simulink model "TestAllDynamicModelsRealForce"  (R2022b)
settings: Solver=FixedStepAuto  StartTime=0.0  StopTime=137  FixedStep=simulator.TimeStep  RelTol=1e-3
undefined symbols (not defined in the file): simulator
settings Model: Creator=At  LastModifiedBy=ateay
settings SolverCC: ConcurrentTasks=on  AlgebraicLoopSolver=TrustRegion  InsertRTBMode=Never (minimum delay)
settings DataIOCC: ReturnWorkspaceOutputs=off
settings DebuggingCC: UnconnectedInputMsg=warning  UnconnectedOutputMsg=warning  UnconnectedLineMsg=warning  SFMachineParentedDataDiag=warning  ArithmeticOperatorsInVariantConditions=warning
settings ModelReferenceCC: EnableRefExpFcnMdlSchedulingChecks=on
settings SFSimCC: SimUseLocalCustomCode=off  CustomCodeUndefinedFunction=UseInterfaceOnly
settings RTWCC: RTWUseLocalCustomCode=off
settings CodeAppCC: StateflowObjectComments=on

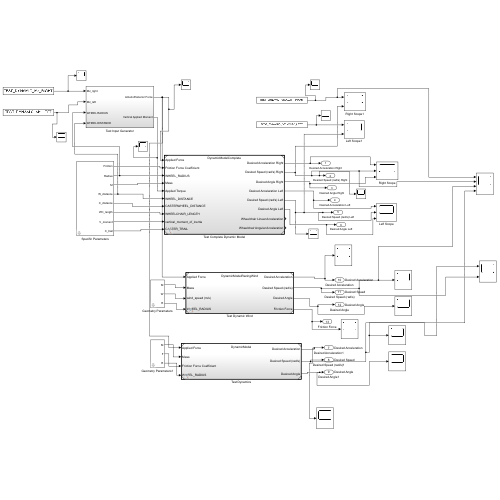
[thumbnail: Simulink's stored preview of the top-level diagram]
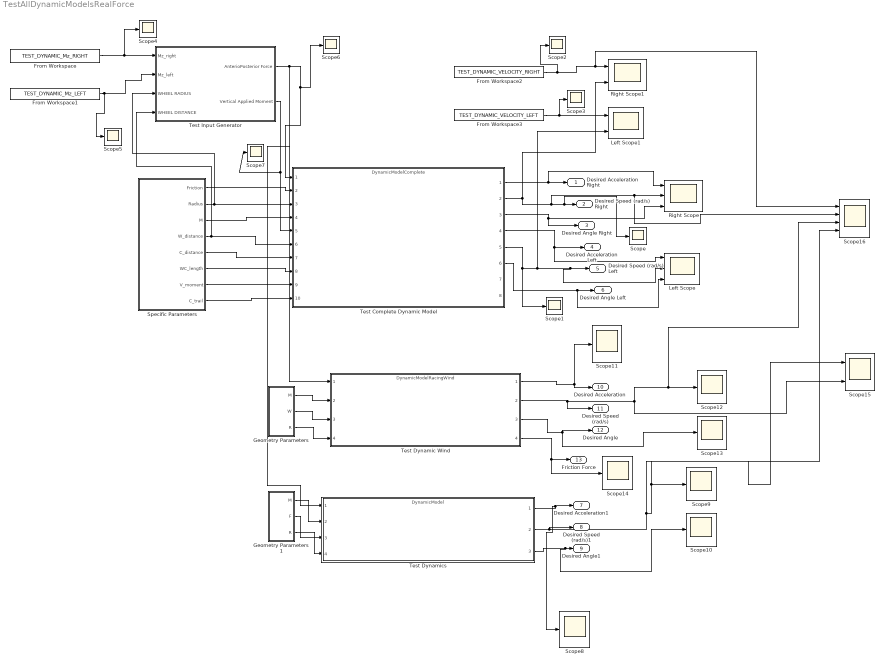
== system TestAllDynamicModelsRealForce ==
  From Workspace : FromWorkspace  VariableName=TEST_DYNAMIC_Mz_RIGHT
  From Workspace1 : FromWorkspace  VariableName=TEST_DYNAMIC_Mz_LEFT
  From Workspace2 : FromWorkspace  VariableName=TEST_DYNAMIC_VELOCITY_RIGHT
  From Workspace3 : FromWorkspace  VariableName=TEST_DYNAMIC_VELOCITY_LEFT
  Geometry Parameters : Subsystem  mask{M=simulator.Sim.Dynamics.Mass, W=simulator.Sim.Dynamics.wind_speed, rR=simulator.Constants.WHEEL_RADIUS}
      mask prompts: M "Mass"; W "Wind"; rR "Radius"
      mask TypeOptions M: Mass/Value
      mask TypeOptions rR: rR/Value
  Geometry Parameters1 : Subsystem  mask{M=simulator.Sim.Dynamics.Mass, F=simulator.Sim.Dynamics.Friction.Coefficient, rR=simulator.Constants.WHEEL_RADIUS}
      mask prompts: M "Mass"; F "Friction"; rR "Radius"
      mask TypeOptions M: Mass/Value
      mask TypeOptions F: Friction/Value
      mask TypeOptions rR: rR/Value
  Left Scope : Scope  NumInputPorts=3
  Left Scope1 : Scope  NumInputPorts=2
  Right Scope : Scope  NumInputPorts=3
  Right Scope1 : Scope  NumInputPorts=2
  Scope{,1..14} (15 alike) : Scope
  Scope15 : Scope  NumInputPorts=2
  Scope16 : Scope  NumInputPorts=4
  Specific Parameters : Subsystem  mask{Friction=simulator.Sim.Dynamics.Friction.Coefficient, Radius=simulator.Constants.WHEEL_RADIUS, M=simulator.Sim.Dynamics.Mass, W_distance=simulator.Constants.WHEEL_DISTANCE, C_distance=simulator.Constants.CASTERWHEEL_DISTANCE, WC_length=simulator.Constants.WHEELCHAIR_LENGTH, V_moment=simulator.Sim.Dynamics.vertical_moment_of_inertia, C_trail=simulator.Constants.CASTER_TRAIL}
      mask prompts: Friction "Friction Force Coefficient"; Radius "WHEEL_RADIUS"; M "Mass"; W_distance "WHEEL_DISTANCE"; C_distance "CASTERWHEEL_DISTANCE"; WC_length "WHEELCHAIR_LENGTH"; V_moment "vertical_moment_of_inertia"; C_trail "CASTER_TRAIL"
  Test Complete Dynamic Model : ModelReference  ModelNameDialog=DynamicModelComplete.slx  SimulationMode=Normal  ModelReferenceVersion=13.2
  Test Dynamic Wind : ModelReference  ModelNameDialog=DynamicModelRacingWind.slx  SimulationMode=Normal  ModelReferenceVersion=1.17
  "Test Dynamics " : ModelReference  ModelNameDialog=DynamicModel.slx  SimulationMode=Normal  ModelReferenceVersion=1.2
  Test Input Generator : Subsystem
  Desired Acceleration Right : Outport
  Desired Speed (rad/s) Right : Outport  Port=2
  Desired Angle Right : Outport  Port=3
  Desired Acceleration Left : Outport  Port=4
  Desired Speed (rad/s) Left : Outport  Port=5
  Desired Angle Left : Outport  Port=6
  Desired Acceleration1 : Outport  Port=7  SignalName=Desired Acceleration
  Desired Speed (rad/s)1 : Outport  Port=8  SignalName=Desired Speed
  Desired Angle1 : Outport  Port=9  SignalName=Desired Angle
  Desired Acceleration : Outport  Port=10  SignalName=Desired Acceleration
  Desired Speed (rad/s) : Outport  Port=11  SignalName=Desired Speed
  Desired Angle : Outport  Port=12  SignalName=Desired Angle
  Friction Force : Outport  Port=13
  wires:
  Test Complete Dynamic Model/1 -> Right Scope/1, Desired Acceleration Right/1
  Test Complete Dynamic Model/2 -> Scope16/2, Right Scope/2, Scope/1, Desired Speed (rad/s) Right/1, Right Scope1/2
  Test Complete Dynamic Model/3 -> Desired Angle Right/1, Right Scope/3
  Test Complete Dynamic Model/5 -> Scope1/1, Left Scope1/2, Left Scope/2, Desired Speed (rad/s) Left/1
  Test Complete Dynamic Model/4 -> Left Scope/1, Desired Acceleration Left/1
  Test Complete Dynamic Model/6 -> Left Scope/3, Desired Angle Left/1
  Specific Parameters/1(Friction) -> Test Complete Dynamic Model/2
  Specific Parameters/2(Radius) -> Test Input Generator/3(WHEEL RADIUS), Test Complete Dynamic Model/3
  Specific Parameters/3(M) -> Test Complete Dynamic Model/4
  Specific Parameters/4(W_distance) -> Test Input Generator/4(WHEEL DISTANCE), Test Complete Dynamic Model/6
  Specific Parameters/5(C_distance) -> Test Complete Dynamic Model/7
  Specific Parameters/6(WC_length) -> Test Complete Dynamic Model/8
  Specific Parameters/7(V_moment) -> Test Complete Dynamic Model/9
  Specific Parameters/8(C_trail) -> Test Complete Dynamic Model/10
  Test Input Generator/1(AnterioPosterior Force) -> "Test Dynamics "/1, Scope6/1, Test Complete Dynamic Model/1, Test Dynamic Wind/1
  Test Input Generator/2(Vertical Applied Moment) -> Scope7/1, Test Complete Dynamic Model/5
  From Workspace/1 -> Scope4/1, Test Input Generator/1(Mz_right)
  From Workspace1/1 -> Scope5/1, Test Input Generator/2(Mz_left)
  From Workspace2/1 -> Scope2/1, Scope16/1, Right Scope1/1
  From Workspace3/1 -> Scope3/1, Left Scope1/1
  Geometry Parameters/1(M) -> Test Dynamic Wind/2
  Geometry Parameters/2(W) -> Test Dynamic Wind/3
  Geometry Parameters/3(R) -> Test Dynamic Wind/4
  Geometry Parameters1/1(M) -> "Test Dynamics "/2
  Geometry Parameters1/2(F) -> "Test Dynamics "/3
  Geometry Parameters1/3(R) -> "Test Dynamics "/4
  "Test Dynamics "/2 -> Desired Speed (rad/s)1/1, Scope16/4, Scope15/1, Scope9/1
  "Test Dynamics "/1 -> Desired Acceleration1/1, Scope8/1
  Test Dynamic Wind/3 -> Desired Angle/1, Scope13/1
  Test Dynamic Wind/2 -> Desired Speed (rad/s)/1, Scope15/2, Scope16/3, Scope12/1
  Test Dynamic Wind/1 -> Desired Acceleration/1, Scope11/1
  Test Dynamic Wind/4 -> Scope14/1, Friction Force/1
  "Test Dynamics "/3 -> Scope10/1, Desired Angle1/1

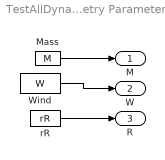
== system TestAllDynamicModelsRealForce/Geometry Parameters ==
  Mass : Constant  Value=M
  Wind : Constant  Value=W
  rR : Constant  Value=rR
  M : Outport
  W : Outport  Port=2
  R : Outport  Port=3
  wires:
  Wind/1 -> W/1
  Mass/1 -> M/1
  rR/1 -> R/1

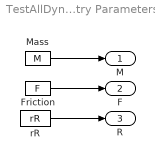
== system TestAllDynamicModelsRealForce/Geometry Parameters1 ==
  Friction : Constant  Value=F
  Mass : Constant  Value=M
  rR : Constant  Value=rR
  M : Outport
  F : Outport  Port=2
  R : Outport  Port=3
  wires:
  Friction/1 -> F/1
  Mass/1 -> M/1
  rR/1 -> R/1

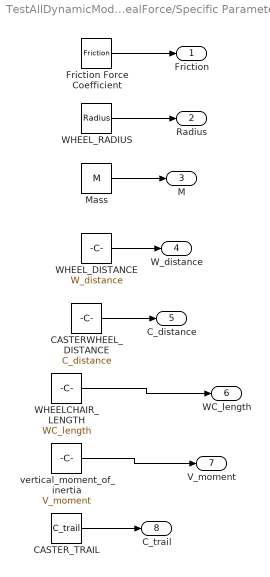
== system TestAllDynamicModelsRealForce/Specific Parameters ==
  CASTERWHEEL_DISTANCE : Constant  Value=C_distance
  CASTER_TRAIL : Constant  Value=C_trail
  Friction Force Coefficient : Constant  Value=Friction
  Mass : Constant  Value=M
  WHEELCHAIR_LENGTH : Constant  Value=WC_length
  WHEEL_DISTANCE : Constant  Value=W_distance
  WHEEL_RADIUS : Constant  Value=Radius
  vertical_moment_of_inertia : Constant  Value=V_moment
  Friction : Outport
  Radius : Outport  Port=2
  M : Outport  Port=3
  W_distance : Outport  Port=4
  C_distance : Outport  Port=5
  WC_length : Outport  Port=6
  V_moment : Outport  Port=7
  C_trail : Outport  Port=8
  wires:
  WHEEL_RADIUS/1 -> Radius/1
  Friction Force Coefficient/1 -> Friction/1
  Mass/1 -> M/1
  CASTERWHEEL_DISTANCE/1 -> C_distance/1
  WHEEL_DISTANCE/1 -> W_distance/1
  WHEELCHAIR_LENGTH/1 -> WC_length/1
  CASTER_TRAIL/1 -> C_trail/1
  vertical_moment_of_inertia/1 -> V_moment/1

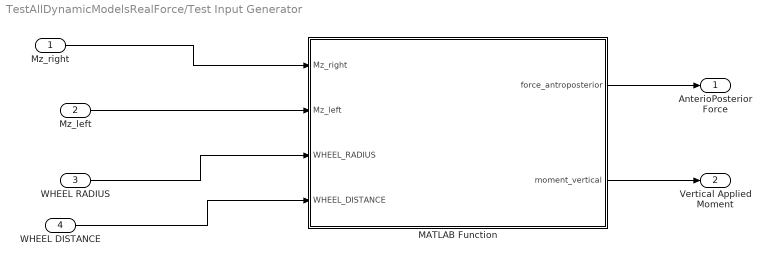
== system TestAllDynamicModelsRealForce/Test Input Generator ==
  Mz_right : Inport
  Mz_left : Inport  Port=2
  WHEEL RADIUS : Inport  Port=3
  WHEEL DISTANCE : Inport  Port=4
  MATLAB Function : MATLAB Function  TreatAsAtomicUnit=on
  AnterioPosterior Force : Outport
  Vertical Applied Moment : Outport  Port=2
  wires:
  Mz_right/1 -> MATLAB Function/1(Mz_right)
  Mz_left/1 -> MATLAB Function/2(Mz_left)
  WHEEL RADIUS/1 -> MATLAB Function/3(WHEEL_RADIUS)
  WHEEL DISTANCE/1 -> MATLAB Function/4(WHEEL_DISTANCE)
  MATLAB Function/1(force_antroposterior) -> AnterioPosterior Force/1
  MATLAB Function/2(moment_vertical) -> Vertical Applied Moment/1

== matlab function TestAllDynamicModelsRealForce/Test Input Generator/MATLAB Function ==
  data: Mz_right input; Mz_left input; WHEEL_RADIUS input; force_antroposterior output; WHEEL_DISTANCE input; moment_vertical output
function [force_antroposterior,moment_vertical]=Force_Conversion(Mz_right, Mz_left,WHEEL_RADIUS,WHEEL_DISTANCE)

%% This function estimates the force and moment applied at the position of installed force cell,...
...based on the moment applied on the right and left instrumented wheels
    
force_antroposterior=(Mz_right/WHEEL_RADIUS)+(Mz_left/WHEEL_RADIUS);
moment_vertical=((Mz_left/WHEEL_RADIUS)-(Mz_right/WHEEL_RADIUS))*(WHEEL_DISTANCE/2);
